simulink model "Quadcopter_Tracking_Final_KCC_2023a"  (R2023a)
settings: Solver=ode5  StartTime=0.0  StopTime=40  FixedStep=0.001  RelTol=1e-3  EnableMultiTasking=on
InitFcn:
  | %Ts = 0.01;
  | %g = 9.81; % gravity constant m/s^2
  | %m = 0.468; % mass of helicopter kg
  | %l = 0.225; % distance between a rotor and the center of quadcopter (m)
  | %k = 2.98e-6; % lift constant
  | %b = 1.14e-7; % drag constant
  | %I_M = 3.357e-5; % rotational moment of inertia kg.m^2
  | % drag force coefficents
  | %A_x = 0.25; % kg/s
  | %A_y = 0.25;
  | %A_z = 0.25;
  | % inertia matrix
  | %I_xx = 4.856e-3; %kgm^2
  | %I_yy = 4.856e-3;
  | %I_zz = 8.801e-3;
  | %KpT = 3.5;
  | %KdT = 4.5;
  | %KpR = 1;
  | %KdR = 3;
undefined symbols (not defined in the file): Ax, Ay, Az, b, g, Ix, Iy, Iz, k, KdR, KdT, KpR, KpT, l, m, Newton, Raphson
settings Model: Creator=Hamed  LastModifiedBy=Admin
settings SolverCC: AlgebraicLoopSolver=TrustRegion
settings DataIOCC: ReturnWorkspaceOutputs=off
settings OptimizationCC: LifeSpan=inf
settings DebuggingCC: MaxConsecutiveZCsMsg=warning  UnconnectedInputMsg=warning  UnconnectedOutputMsg=warning  UnconnectedLineMsg=warning  SFUnexpectedBacktrackingDiag=warning  SFNoUnconditionalDefaultTransitionDiag=warning  SFExecutionAtInitializationDiag=none  ArithmeticOperatorsInVariantConditions=warning
settings HardwareCC: ProdBitPerSizeT=32  ProdBitPerPtrDiffT=32  ProdWordSize=32  ProdHWDeviceType=Specified
settings ModelReferenceCC: EnableRefExpFcnMdlSchedulingChecks=on
settings SFSimCC: SimUseLocalCustomCode=off  CustomCodeUndefinedFunction=UseInterfaceOnly
settings RTWCC: RTWUseLocalCustomCode=off  DLArmComputeVersion=19.05
settings CodeAppCC: StateflowObjectComments=on
settings GRTTargetCC: TargetLangStandard=C89/C90 (ANSI)
settings ConfigComp: CovMetricSettings=dw  CovSaveCumulativeToWorkspaceVar=on  CovSaveSingleToWorkspaceVar=on  CovExternalEMLEnable=off

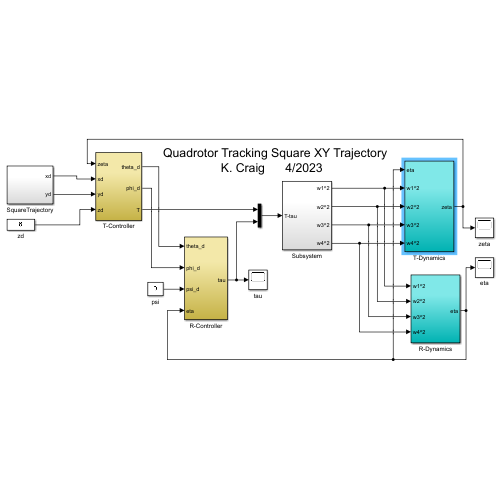
[thumbnail: Simulink's stored preview of the top-level diagram]
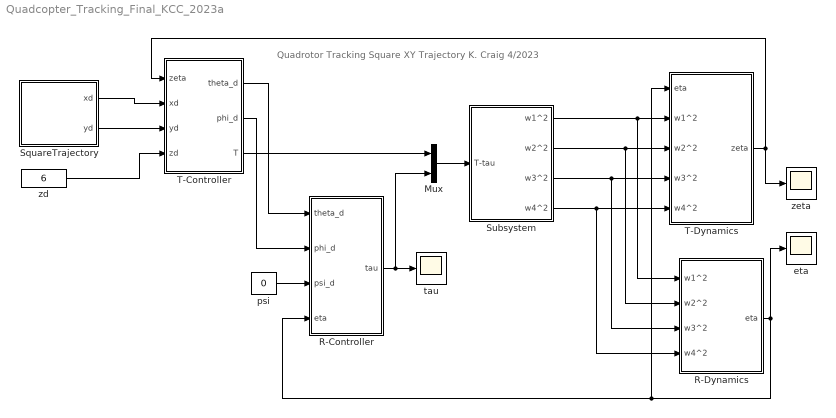
== system Quadcopter_Tracking_Final_KCC_2023a ==
  note: Quadrotor Tracking Square XY Trajectory
      | K. Craig 4/2023
  Mux : Mux  Inputs=2
  R-Controller : Subsystem
  R-Dynamics : Subsystem
  SquareTrajectory : Subsystem
  Subsystem : Subsystem
  T-Controller : Subsystem
  T-Dynamics : Subsystem
  eta : Scope
  psi : Constant  Value=0
  tau : Scope
  zd : Constant  Value=6
  zeta : Scope
  wires:
  T-Dynamics/1(zeta) -> zeta/1, T-Controller/1(zeta)
  R-Dynamics/1(eta) -> T-Dynamics/1(eta), R-Controller/4(eta), eta/1
  psi/1 -> R-Controller/3(psi_d)
  zd/1 -> T-Controller/4(zd)
  T-Controller/1(theta_d) -> R-Controller/1(theta_d)
  T-Controller/2(phi_d) -> R-Controller/2(phi_d)
  T-Controller/3(T) -> Mux/1
  R-Controller/1(tau) -> tau/1, Mux/2
  Mux/1 -> Subsystem/1(T-tau)
  Subsystem/1(w1^2) -> R-Dynamics/1(w1^2), T-Dynamics/2(w1^2)
  Subsystem/2(w2^2) -> R-Dynamics/2(w2^2), T-Dynamics/3(w2^2)
  Subsystem/3(w3^2) -> T-Dynamics/4(w3^2), R-Dynamics/3(w3^2)
  Subsystem/4(w4^2) -> R-Dynamics/4(w4^2), T-Dynamics/5(w4^2)
  SquareTrajectory/1(xd) -> T-Controller/2(xd)
  SquareTrajectory/2(yd) -> T-Controller/3(yd)

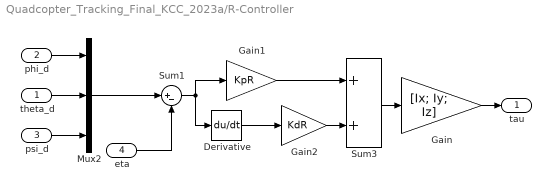
== system Quadcopter_Tracking_Final_KCC_2023a/R-Controller ==
  theta_d : Inport
  phi_d : Inport  Port=2
  psi_d : Inport  Port=3
  eta : Inport  Port=4
  Derivative : Derivative
  Gain : Gain  Gain=[Ix; Iy; Iz]
  Gain1 : Gain  Gain=KpR
  Gain2 : Gain  Gain=KdR
  Mux2 : Mux  Inputs=3
  Sum1 : Sum  Inputs=|+-
  Sum3 : Sum
  tau : Outport
  wires:
  eta/1 -> Sum1/2
  phi_d/1 -> Mux2/1
  theta_d/1 -> Mux2/2
  psi_d/1 -> Mux2/3
  Gain/1 -> tau/1
  Gain2/1 -> Sum3/2
  Gain1/1 -> Sum3/1
  Derivative/1 -> Gain2/1
  Sum1/1 -> Derivative/1, Gain1/1
  Sum3/1 -> Gain/1
  Mux2/1 -> Sum1/1

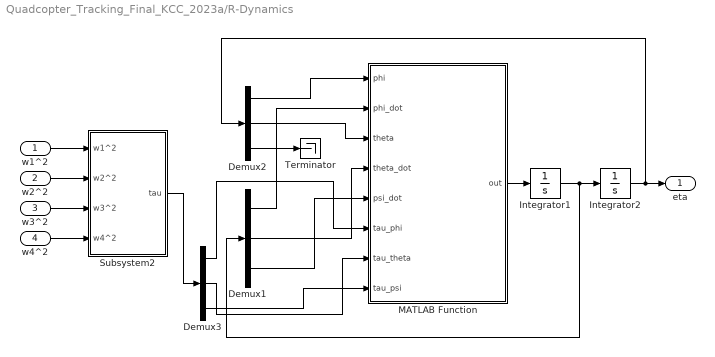
== system Quadcopter_Tracking_Final_KCC_2023a/R-Dynamics ==
  w1^2 : Inport
  w2^2 : Inport  Port=2
  w3^2 : Inport  Port=3
  w4^2 : Inport  Port=4
  Demux1 : Demux  Outputs=3
  Demux2 : Demux  Outputs=3
  Demux3 : Demux  Outputs=3
  Integrator1 : Integrator  IgnoreLimit=on
  Integrator2 : Integrator  InitialCondition=[0; 0; 0]
  MATLAB Function : MATLAB Function  TreatAsAtomicUnit=on
  Subsystem2 : Subsystem
  Terminator : Terminator
  eta : Outport
  wires:
  Integrator1/1 -> Demux1/1, Integrator2/1
  Integrator2/1 -> Demux2/1, eta/1
  w2^2/1 -> Subsystem2/2(w2^2)
  w4^2/1 -> Subsystem2/4(w4^2)
  w1^2/1 -> Subsystem2/1(w1^2)
  w3^2/1 -> Subsystem2/3(w3^2)
  Demux2/3 -> Terminator/1
  MATLAB Function/1(out) -> Integrator1/1
  Demux2/1 -> MATLAB Function/1(phi)
  Demux2/2 -> MATLAB Function/3(theta)
  Demux1/1 -> MATLAB Function/2(phi_dot)
  Demux1/2 -> MATLAB Function/4(theta_dot)
  Demux1/3 -> MATLAB Function/5(psi_dot)
  Subsystem2/1(tau) -> Demux3/1
  Demux3/1 -> MATLAB Function/6(tau_phi)
  Demux3/2 -> MATLAB Function/7(tau_theta)
  Demux3/3 -> MATLAB Function/8(tau_psi)

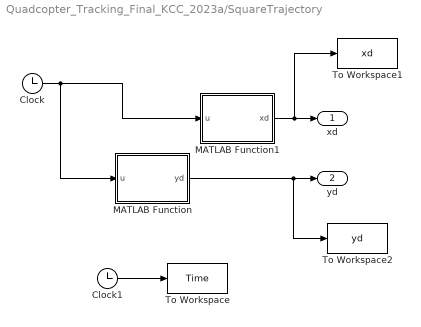
== system Quadcopter_Tracking_Final_KCC_2023a/SquareTrajectory ==
  Clock : Clock
  Clock1 : Clock
  MATLAB Function : MATLAB Function  TreatAsAtomicUnit=on
  MATLAB Function1 : MATLAB Function  TreatAsAtomicUnit=on
  To Workspace : ToWorkspace  VariableName=Time  SampleTime=-1
  To Workspace1 : ToWorkspace  VariableName=xd  SampleTime=-1
  To Workspace2 : ToWorkspace  VariableName=yd  SampleTime=-1
  xd : Outport
  yd : Outport  Port=2
  wires:
  MATLAB Function/1(yd) -> To Workspace2/1, yd/1
  MATLAB Function1/1(xd) -> To Workspace1/1, xd/1
  Clock/1 -> MATLAB Function/1(u), MATLAB Function1/1(u)
  Clock1/1 -> To Workspace/1

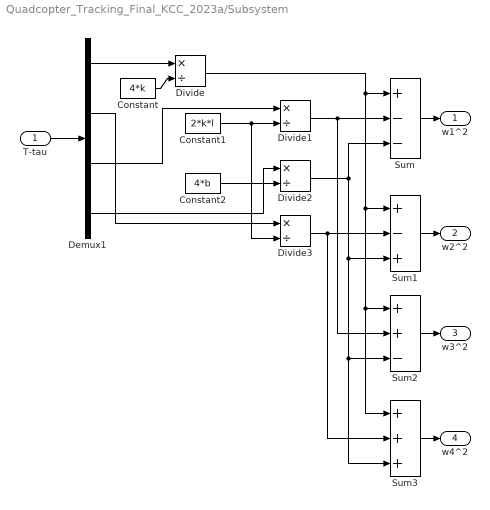
== system Quadcopter_Tracking_Final_KCC_2023a/Subsystem ==
  T-tau : Inport
  Constant : Constant  Value=4*k
  Constant1 : Constant  Value=2*k*l
  Constant2 : Constant  Value=4*b
  Demux1 : Demux
  Divide{,1..3} (4 alike) : Product  Inputs=*/
  Sum : Sum  Inputs=+--
  Sum1 : Sum  Inputs=+-+
  Sum2 : Sum  Inputs=++-
  Sum3 : Sum  Inputs=+++
  w1^2 : Outport
  w2^2 : Outport  Port=2
  w3^2 : Outport  Port=3
  w4^2 : Outport  Port=4
  wires:
  Sum1/1 -> w2^2/1
  T-tau/1 -> Demux1/1
  Sum3/1 -> w4^2/1
  Sum/1 -> w1^2/1
  Demux1/2 -> Divide3/1
  Divide3/1 -> Sum3/2, Sum1/2
  Sum2/1 -> w3^2/1
  Constant/1 -> Divide/2
  Constant2/1 -> Divide2/2
  Demux1/1 -> Divide/1
  Demux1/3 -> Divide1/1
  Demux1/4 -> Divide2/1
  Constant1/1 -> Divide3/2, Divide1/2
  Divide/1 -> Sum3/1, Sum2/1, Sum1/1, Sum/1
  Divide2/1 -> Sum/3, Sum3/3, Sum2/3, Sum1/3
  Divide1/1 -> Sum2/2, Sum/2

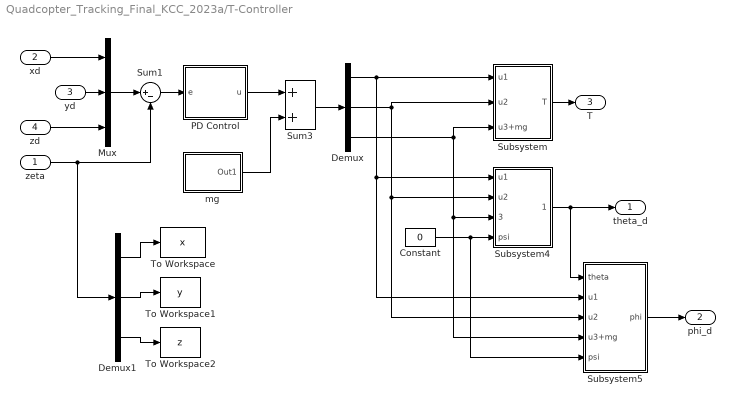
== system Quadcopter_Tracking_Final_KCC_2023a/T-Controller ==
  zeta : Inport
  xd : Inport  Port=2
  yd : Inport  Port=3
  zd : Inport  Port=4
  Constant : Constant  Value=0
  Demux : Demux  Outputs=3
  Demux1 : Demux  Outputs=3
  Mux : Mux  Inputs=3
  PD Control : Subsystem
  Subsystem : Subsystem
  Subsystem4 : Subsystem
  Subsystem5 : Subsystem
  Sum1 : Sum  Inputs=|+-
  Sum3 : Sum
  To Workspace : ToWorkspace  VariableName=x  SampleTime=-1
  To Workspace1 : ToWorkspace  VariableName=y  SampleTime=-1
  To Workspace2 : ToWorkspace  VariableName=z  SampleTime=-1
  mg : Subsystem
  theta_d : Outport
  phi_d : Outport  Port=2
  T : Outport  Port=3
  wires:
  Subsystem4/1(theta) -> Subsystem5/1(theta), theta_d/1
  Subsystem/1(T) -> T/1
  Subsystem5/1(phi) -> phi_d/1
  Constant/1 -> Subsystem4/4(psi), Subsystem5/5(psi)
  xd/1 -> Mux/1
  yd/1 -> Mux/2
  zd/1 -> Mux/3
  Demux/1 -> Subsystem5/2(u1), Subsystem4/1(u1), Subsystem/1(u1)
  Demux/2 -> Subsystem5/3(u2), Subsystem4/2(u2), Subsystem/2(u2)
  Demux/3 -> Subsystem5/4(u3+mg), Subsystem4/3(u3+mg), Subsystem/3(u3+mg)
  Mux/1 -> Sum1/1
  zeta/1 -> Demux1/1, Sum1/2
  mg/1(Out1) -> Sum3/2
  Sum1/1 -> PD Control/1(e)
  PD Control/1(u) -> Sum3/1
  Sum3/1 -> Demux/1
  Demux1/1 -> To Workspace/1
  Demux1/2 -> To Workspace1/1
  Demux1/3 -> To Workspace2/1

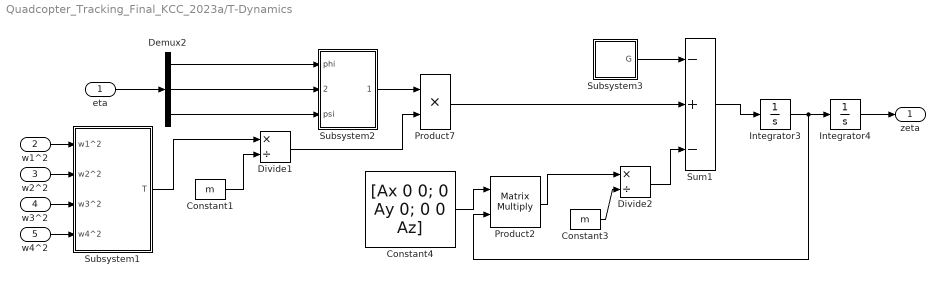
== system Quadcopter_Tracking_Final_KCC_2023a/T-Dynamics ==
  eta : Inport
  w1^2 : Inport  Port=2
  w2^2 : Inport  Port=3
  w3^2 : Inport  Port=4
  w4^2 : Inport  Port=5
  Constant1 : Constant  Value=m
  Constant3 : Constant  Value=m
  Constant4 : Constant  Value=[Ax 0 0; 0 Ay 0; 0 0 Az]
  Demux2 : Demux  Outputs=3
  Divide1 : Product  Inputs=*/
  Divide2 : Product  Inputs=*/
  Integrator3 : Integrator
  Integrator4 : Integrator  InitialCondition=[0; 0; 2]
  Product2 : Product  Multiplication=Matrix(*)
  Product7 : Product
  Subsystem1 : Subsystem
  Subsystem2 : Subsystem
  Subsystem3 : Subsystem
  Sum1 : Sum  Inputs=-+-
  zeta : Outport
  wires:
  Subsystem2/1(Out1) -> Product7/1
  Constant4/1 -> Product2/1
  Subsystem3/1(G) -> Sum1/1
  Integrator3/1 -> Product2/2, Integrator4/1
  Sum1/1 -> Integrator3/1
  Subsystem1/1(T) -> Divide1/1
  Product7/1 -> Sum1/2
  Product2/1 -> Divide2/1
  Integrator4/1 -> zeta/1
  Constant1/1 -> Divide1/2
  Divide1/1 -> Product7/2
  Constant3/1 -> Divide2/2
  Divide2/1 -> Sum1/3
  eta/1 -> Demux2/1
  Demux2/1 -> Subsystem2/1(phi)
  Demux2/2 -> Subsystem2/2(theta)
  Demux2/3 -> Subsystem2/3(psi)
  w1^2/1 -> Subsystem1/1(w1^2)
  w2^2/1 -> Subsystem1/2(w2^2)
  w3^2/1 -> Subsystem1/3(w3^2)
  w4^2/1 -> Subsystem1/4(w4^2)

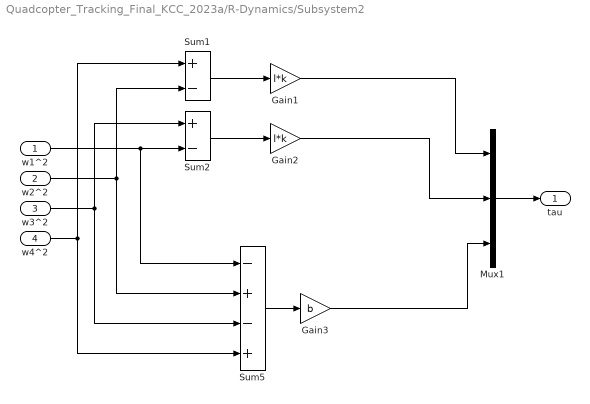
== system Quadcopter_Tracking_Final_KCC_2023a/R-Dynamics/Subsystem2 ==
  w1^2 : Inport
  w2^2 : Inport  Port=2
  w3^2 : Inport  Port=3
  w4^2 : Inport  Port=4
  Gain1 : Gain  Gain=l*k
  Gain2 : Gain  Gain=l*k
  Gain3 : Gain  Gain=b
  Mux1 : Mux  Inputs=3
  Sum1 : Sum  Inputs=+-
  Sum2 : Sum  Inputs=+-
  Sum5 : Sum  Inputs=-+-+
  tau : Outport
  wires:
  Gain1/1 -> Mux1/1
  Gain3/1 -> Mux1/3
  Gain2/1 -> Mux1/2
  Sum2/1 -> Gain2/1
  w1^2/1 -> Sum5/1, Sum2/2
  w2^2/1 -> Sum1/2, Sum5/2
  Sum1/1 -> Gain1/1
  w4^2/1 -> Sum1/1, Sum5/4
  w3^2/1 -> Sum2/1, Sum5/3
  Mux1/1 -> tau/1
  Sum5/1 -> Gain3/1

== system Quadcopter_Tracking_Final_KCC_2023a/T-Controller/PD Control ==
  e : Inport
  Derivative : Derivative
  Gain : Gain  Gain=KpT
  Gain1 : Gain  Gain=KdT
  Sum2 : Sum
  u : Outport
  wires:
  Gain/1 -> Sum2/1
  e/1 -> Gain/1, Derivative/1
  Derivative/1 -> Gain1/1
  Gain1/1 -> Sum2/2
  Sum2/1 -> u/1

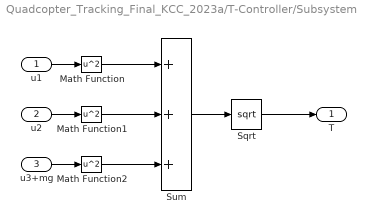
== system Quadcopter_Tracking_Final_KCC_2023a/T-Controller/Subsystem ==
  u1 : Inport
  u2 : Inport  Port=2
  u3+mg : Inport  Port=3
  Math Function : Math  Operator=square
  Math Function1 : Math  Operator=square
  Math Function2 : Math  Operator=square
  Sqrt : Sqrt  AlgorithmType=Newton-Raphson
  Sum : Sum  Inputs=+++
  T : Outport
  wires:
  Sqrt/1 -> T/1
  Math Function/1 -> Sum/1
  Math Function1/1 -> Sum/2
  Math Function2/1 -> Sum/3
  Sum/1 -> Sqrt/1
  u1/1 -> Math Function/1
  u2/1 -> Math Function1/1
  u3+mg/1 -> Math Function2/1

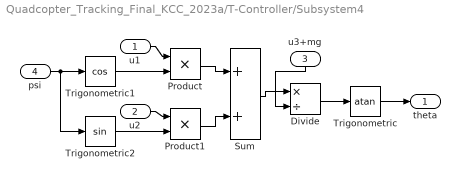
== system Quadcopter_Tracking_Final_KCC_2023a/T-Controller/Subsystem4 ==
  u1 : Inport
  u2 : Inport  Port=2
  u3+mg : Inport  Port=3
  psi : Inport  Port=4
  Divide : Product  Inputs=*/
  Product : Product  RndMeth=Zero
  Product1 : Product  RndMeth=Zero
  Sum : Sum
  Trigonometric : Trigonometry  Operator=atan
  Trigonometric1 : Trigonometry  Operator=cos
  Trigonometric2 : Trigonometry
  theta : Outport
  wires:
  Trigonometric1/1 -> Product/2
  Trigonometric2/1 -> Product1/2
  Product/1 -> Sum/1
  Product1/1 -> Sum/2
  Sum/1 -> Divide/1
  Divide/1 -> Trigonometric/1
  u1/1 -> Product/1
  u3+mg/1 -> Divide/2
  u2/1 -> Product1/1
  Trigonometric/1 -> theta/1
  psi/1 -> Trigonometric1/1, Trigonometric2/1

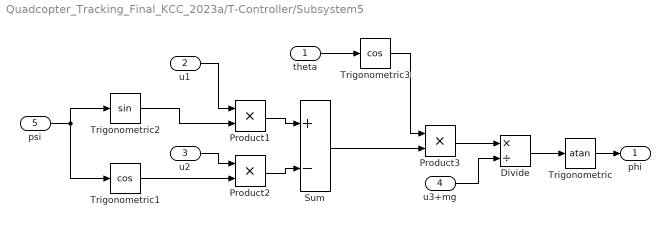
== system Quadcopter_Tracking_Final_KCC_2023a/T-Controller/Subsystem5 ==
  theta : Inport
  u1 : Inport  Port=2
  u2 : Inport  Port=3
  u3+mg : Inport  Port=4
  psi : Inport  Port=5
  Divide : Product  Inputs=*/
  Product1 : Product  RndMeth=Zero
  Product2 : Product  RndMeth=Zero
  Product3 : Product  RndMeth=Zero
  Sum : Sum  Inputs=+-
  Trigonometric : Trigonometry  Operator=atan
  Trigonometric1 : Trigonometry  Operator=cos
  Trigonometric2 : Trigonometry
  Trigonometric3 : Trigonometry  Operator=cos
  phi : Outport
  wires:
  Trigonometric2/1 -> Product1/2
  Trigonometric1/1 -> Product2/2
  Product1/1 -> Sum/1
  Product2/1 -> Sum/2
  Sum/1 -> Product3/2
  Trigonometric3/1 -> Product3/1
  Product3/1 -> Divide/1
  Divide/1 -> Trigonometric/1
  psi/1 -> Trigonometric2/1, Trigonometric1/1
  u1/1 -> Product1/1
  u2/1 -> Product2/1
  theta/1 -> Trigonometric3/1
  Trigonometric/1 -> phi/1
  u3+mg/1 -> Divide/2

== system Quadcopter_Tracking_Final_KCC_2023a/T-Controller/mg ==
  Constant1 : Constant  Value=m*g
  Constant2 : Constant  Value=0
  Mux1 : Mux  Inputs=3
  Out1 : Outport
  wires:
  Mux1/1 -> Out1/1
  Constant1/1 -> Mux1/3
  Constant2/1 -> Mux1/2, Mux1/1

== system Quadcopter_Tracking_Final_KCC_2023a/T-Dynamics/Subsystem1 ==
  w1^2 : Inport
  w2^2 : Inport  Port=2
  w3^2 : Inport  Port=3
  w4^2 : Inport  Port=4
  Gain : Gain  Gain=k
  Sum : Sum  Inputs=++++
  T : Outport
  wires:
  w1^2/1 -> Sum/1
  Sum/1 -> Gain/1
  w2^2/1 -> Sum/2
  w4^2/1 -> Sum/4
  w3^2/1 -> Sum/3
  Gain/1 -> T/1

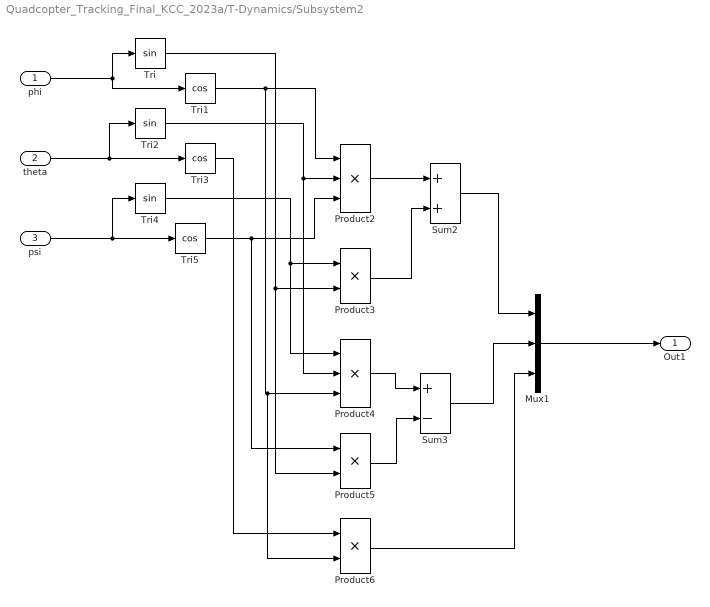
== system Quadcopter_Tracking_Final_KCC_2023a/T-Dynamics/Subsystem2 ==
  phi : Inport
  theta : Inport  Port=2
  psi : Inport  Port=3
  Mux1 : Mux  Inputs=3
  Product2 : Product  Inputs=3
  Product3 : Product
  Product4 : Product  Inputs=3
  Product5 : Product
  Product6 : Product
  Sum2 : Sum
  Sum3 : Sum  Inputs=+-
  Tri : Trigonometry
  Tri1 : Trigonometry  Operator=cos
  Tri2 : Trigonometry
  Tri3 : Trigonometry  Operator=cos
  Tri4 : Trigonometry
  Tri5 : Trigonometry  Operator=cos
  Out1 : Outport
  wires:
  Tri4/1 -> Product4/1, Product3/1
  Tri/1 -> Product5/2, Product3/2
  Product3/1 -> Sum2/2
  Tri1/1 -> Product6/2, Product4/3, Product2/1
  Product2/1 -> Sum2/1
  Sum2/1 -> Mux1/1
  phi/1 -> Tri/1, Tri1/1
  Product6/1 -> Mux1/3
  theta/1 -> Tri2/1, Tri3/1
  Product4/1 -> Sum3/1
  Tri2/1 -> Product4/2, Product2/2
  Product5/1 -> Sum3/2
  psi/1 -> Tri4/1, Tri5/1
  Tri5/1 -> Product5/1, Product2/3
  Mux1/1 -> Out1/1
  Tri3/1 -> Product6/1
  Sum3/1 -> Mux1/2

== system Quadcopter_Tracking_Final_KCC_2023a/T-Dynamics/Subsystem3 ==
  Constant : Constant  Value=0
  Constant1 : Constant  Value=g
  Mux : Mux  Inputs=3
  G : Outport
  wires:
  Mux/1 -> G/1
  Constant1/1 -> Mux/3
  Constant/1 -> Mux/2, Mux/1

== matlab function Quadcopter_Tracking_Final_KCC_2023a/R-Dynamics/MATLAB Function ==
  data: phi input; out output; phi_dot input; theta input; theta_dot input; psi_dot input; tau_phi input; tau_theta input; tau_psi input
function out  = quadcopter(phi, phi_dot, theta, theta_dot, psi_dot, tau_phi, tau_theta, tau_psi)

% Quadcopter Parameters (SI Units)

Ix = 4.856E-3;
Iy = 4.856E-3;
Iz = 8.801E-3;

m = 0.468;
l = 0.225;
g = 9.81;
k = 2.980E-6;
b = 1.140E-7;
psi = 0;

% eta =[phi theta psi]'
% J*eta_ddot + C*eta_dot = [tau_phi tau_theta tau_psi]'

J = zeros(3,3);
C = zeros(3,3);

J(1,1) = Ix;
J(1,2) = 0;
J(1,3) = -Ix*sin(theta);
J(2,1) = 0;
J(2,2) = Iy*(cos(phi))^2 + Iz*(sin(phi))^2;
J(2,3) = (Iy-Iz)*cos(phi)*sin(phi)*cos(theta);
J(3,1) = -Ix*sin(theta);
J(3,2) = (Iy-Iz)*cos(phi)*sin(phi)*cos(theta);
J(3,3) = Ix*(sin(theta))^2 + Iy*(sin(phi))^2*(cos(theta))^2 + Iz*(cos(phi))^2*(cos(theta))^2;

C(1,1) = 0;
C(1,2) = (Iy-Iz)*(theta_dot*cos(phi)*sin(phi)+psi_dot*(sin(phi))^2*cos(theta))+...
    (Iz-Iy)*psi_dot*(cos(phi))^2*cos(theta)-Ix*psi_dot*cos(theta);
C(1,3) = (Iz-Iy)*psi_dot*cos(phi)*sin(phi)*(cos(theta))^2;
C(2,1) =  (Iz-Iy)*(theta_dot*cos(phi)*sin(phi)+psi_dot*sin(phi)*cos(theta))+...
    (Iy-Iz)*psi_dot*(cos(phi))^2*cos(theta)+Ix*psi_dot*cos(theta);
C(2,2) = (Iz-Iy)*phi_dot*cos(phi)*sin(phi);
C(2,3) = -Ix*psi_dot*sin(theta)*cos(theta)+Iy*psi_dot*(sin(phi))^2*sin(theta)*cos(theta)+...
    Iz*psi_dot*(cos(phi))^2*sin(theta)*cos(theta);
C(3,1) = (Iy-Iz)*psi_dot*(cos(theta))^2*sin(phi)*cos(phi)-Ix*theta_dot*cos(theta);
C(3,2) = (Iz-Iy)*(theta_dot*cos(phi)*sin(phi)*sin(theta)+phi_dot*(sin(phi))^2*cos(theta))+...
    (Iy-Iz)*phi_dot*(cos(phi))^2*cos(theta)+Ix*psi_dot*sin(theta)*cos(theta)-...
    Iy*psi_dot*(sin(phi))^2*sin(theta)*cos(theta)-Iz*psi_dot*(cos(phi))^2*sin(theta)*cos(theta);
C(3,3) = (Iy-Iz)*phi_dot*cos(phi)*sin(phi)*(cos(theta))^2-Iy*theta_dot*(sin(phi))^2*cos(theta)*sin(theta)-...
    Iz*theta_dot*(cos(phi))^2*cos(theta)*sin(theta)+Ix*theta_dot*cos(theta)*sin(theta);

B = [tau_phi tau_theta tau_psi]';

N = [phi_dot theta_dot psi_dot]';

out = [inv(J)*(B-C*N)];
end

== matlab function Quadcopter_Tracking_Final_KCC_2023a/SquareTrajectory/MATLAB Function ==
  data: u input; yd output
function yd = fcn(u)
%#codegen
yd = 0;
if u < 10
    yd = u;
end
if u>=10 && u<20
    yd = 10;
end
if u>=20 && u<30
    yd = 30 - u;
end
if u>=30 && u<40
    yd = 0;
end

== matlab function Quadcopter_Tracking_Final_KCC_2023a/SquareTrajectory/MATLAB Function1 ==
  data: u input; xd output
function xd = fcn(u)
%#codegen
xd = 0;
if u < 10
    xd = 0;
end
if u>=10 && u<20
    xd = -10 + u;
end
if u>=20 && u<30
    xd = 10;
end
if u>=30 && u<40
    xd = 40 - u;
end
